simulink model "nominal_model_sliding_mode"  (R2019b)
settings: Solver=VariableStepAuto  StartTime=0.0  StopTime=10.0  RelTol=1e-3
settings Model: Creator=Alien  LastModifiedBy=Alien
settings DebuggingCC: UnderSpecifiedDimensionMsg=warning

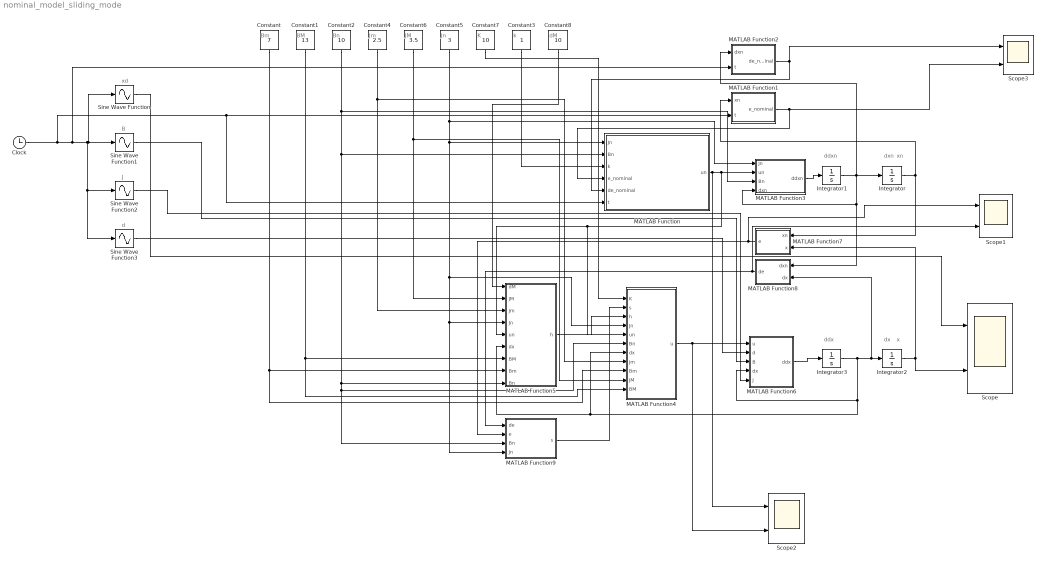
== system nominal_model_sliding_mode ==
  note: xd
  note: Bm
  note: ddxn
  note: dxn
  note: xn
  note: x
  note: dx
  note: ddx
  note: BM
  note: Bn
  note: Jm
  note: Jn
  note: JM
  note: K
  note: k
  note: dM
  note: B
  note: J
  note: d
  Clock : Clock
  Constant : Constant  Value=7
  Constant1 : Constant  Value=13
  Constant2 : Constant  Value=10
  Constant3 : Constant
  Constant4 : Constant  Value=2.5
  Constant5 : Constant  Value=3
  Constant6 : Constant  Value=3.5
  Constant7 : Constant  Value=10
  Constant8 : Constant  Value=10
  Integrator{,1..3} (4 alike) : Integrator
  MATLAB Function : MATLAB Function  TreatAsAtomicUnit=on
  MATLAB Function1 : MATLAB Function  TreatAsAtomicUnit=on
  MATLAB Function2 : MATLAB Function  TreatAsAtomicUnit=on
  MATLAB Function3 : MATLAB Function  TreatAsAtomicUnit=on
  MATLAB Function4 : MATLAB Function  TreatAsAtomicUnit=on
  MATLAB Function5 : MATLAB Function  TreatAsAtomicUnit=on
  MATLAB Function6 : MATLAB Function  TreatAsAtomicUnit=on
  MATLAB Function7 : MATLAB Function  TreatAsAtomicUnit=on
  MATLAB Function8 : MATLAB Function  TreatAsAtomicUnit=on
  MATLAB Function9 : MATLAB Function  TreatAsAtomicUnit=on
  Scope{,1..3} (4 alike) : Scope  NumInputPorts=2
  Sine Wave Function : Sin  TimeSource=Use external signal  SampleTime=0
  Sine Wave Function1 : Sin  TimeSource=Use external signal  Amplitude=3  Bias=10  Frequency=2*pi  SampleTime=0
  Sine Wave Function2 : Sin  TimeSource=Use external signal  Amplitude=0.5  Bias=3  Frequency=2*pi  SampleTime=0
  Sine Wave Function3 : Sin  TimeSource=Use external signal  Amplitude=10  SampleTime=0
  wires:
  MATLAB Function3/1(ddxn) -> Integrator1/1
  MATLAB Function/1(un) -> Scope2/1, MATLAB Function4/5(un), MATLAB Function5/5(un), MATLAB Function3/2(un)
  Integrator1/1 -> MATLAB Function8/1(dxn), MATLAB Function3/4(dxn), MATLAB Function2/1(dxn), Integrator/1
  Integrator/1 -> MATLAB Function7/1(xn), MATLAB Function1/1(xn)
  MATLAB Function2/1(de_nominal) -> Scope3/1, MATLAB Function/5(de_nominal)
  MATLAB Function1/1(e_nominal) -> Scope3/2, MATLAB Function/4(e_nominal)
  MATLAB Function5/1(h) -> MATLAB Function4/3(h)
  MATLAB Function4/1(u) -> Scope2/2, MATLAB Function6/1(u)
  Integrator3/1 -> MATLAB Function8/2(dx), Integrator2/1, MATLAB Function6/4(dx), MATLAB Function4/7(dx), MATLAB Function5/6(dx)
  MATLAB Function6/1(ddx) -> Integrator3/1
  Integrator2/1 -> Scope/2, MATLAB Function7/2(x)
  Constant7/1 -> MATLAB Function4/1(K)
  Constant8/1 -> MATLAB Function5/1(dM)
  Constant6/1 -> MATLAB Function4/10(JM), MATLAB Function5/2(JM)
  Constant4/1 -> MATLAB Function4/8(Jm), MATLAB Function5/3(Jm)
  Constant5/1 -> MATLAB Function3/1(Jn), MATLAB Function/1(Jn), MATLAB Function4/4(Jn), MATLAB Function9/4(Jn), MATLAB Function5/4(Jn)
  Constant1/1 -> MATLAB Function4/11(BM), MATLAB Function5/7(BM)
  Constant/1 -> MATLAB Function4/9(Bm), MATLAB Function5/8(Bm)
  Constant2/1 -> MATLAB Function/2(Bn), MATLAB Function4/6(Bn), MATLAB Function9/3(Bn), MATLAB Function5/9(Bn), MATLAB Function3/3(Bn)
  Constant3/1 -> MATLAB Function/3(k)
  Clock/1 -> MATLAB Function/6(t), MATLAB Function1/2(t), MATLAB Function2/2(t), Sine Wave Function3/1, Sine Wave Function2/1, Sine Wave Function/1, Sine Wave Function1/1
  Sine Wave Function1/1 -> MATLAB Function6/3(B)
  Sine Wave Function2/1 -> MATLAB Function6/5(J)
  Sine Wave Function3/1 -> MATLAB Function6/2(d)
  MATLAB Function7/1(e) -> Scope1/1, MATLAB Function9/2(e)
  MATLAB Function8/1(de) -> MATLAB Function9/1(de), Scope1/2
  MATLAB Function9/1(s) -> MATLAB Function4/2(s)
  Sine Wave Function/1 -> Scope/1

== matlab function nominal_model_sliding_mode/MATLAB Function1 ==
  data: xn input; e_nominal output; t input
function e_nominal = fcn(xn, t)
e_nominal = xn - sin(t);

== matlab function nominal_model_sliding_mode/MATLAB Function ==
  data: Jn input; un output; Bn input; k input; e_nominal input; de_nominal input; t input
function un = fcn(Jn, Bn, k, e_nominal, de_nominal, t)
h1 = k^2;
h2 = 2*k - Bn/Jn;
dthet_d = cos(t);
ddthet_d = -sin(t);
un = Jn*(Bn/Jn*dthet_d + ddthet_d - h1*e_nominal - h2*de_nominal);

== matlab function nominal_model_sliding_mode/MATLAB Function2 ==
  data: dxn input; de_nominal output; t input
function de_nominal = fcn(dxn, t)
de_nominal = dxn - cos(t);

== matlab function nominal_model_sliding_mode/MATLAB Function3 ==
  data: Jn input; ddxn output; un input; Bn input; dxn input
function ddxn = fcn(Jn, un, Bn, dxn)
ddxn = 1/Jn*(un - Bn*dxn);

== matlab function nominal_model_sliding_mode/MATLAB Function4 ==
  data: K input; u output; s input; h input; Jn input; un input; Bn input; dx input; Jm input; Bm input; JM input; BM input
function u = fcn(K, s, h, Jn, un, Bn, dx, Jm, Bm, JM, BM)
lamd = Bn/Jn;
Ja = (Jm + JM)/2;
Ba = (Bm + BM)/2;
u = -K*s - h*sign(s) + Ja*(1/Jn*un - lamd*dx) + Ba*dx;

== matlab function nominal_model_sliding_mode/MATLAB Function5 ==
  data: dM input; h output; JM input; Jm input; Jn input; un input; dx input; BM input; Bm input; Bn input
function h = fcn(dM, JM, Jm, Jn, un, dx, BM, Bm, Bn)
lamd = Bn/Jn;
h = dM + (JM - Jm)*abs(1/Jn*un - lamd*dx)/2 + (BM - Bm)*abs(dx)/2;

== matlab function nominal_model_sliding_mode/MATLAB Function6 ==
  data: u input; ddx output; d input; B input; dx input; J input
function ddx = fcn(u, d, B, dx, J)
ddx = 1/J*(u - d - B*dx);

== matlab function nominal_model_sliding_mode/MATLAB Function7 ==
  data: xn input; e output; x input
function e = fcn(xn, x)
e = x - xn;

== matlab function nominal_model_sliding_mode/MATLAB Function8 ==
  data: dxn input; de output; dx input
function de = fcn(dxn, dx)
de = dx - dxn;

== matlab function nominal_model_sliding_mode/MATLAB Function9 ==
  data: de input; s output; e input; Bn input; Jn input
function s = fcn(de, e, Bn, Jn)
s = de + Bn/Jn*e;
